simulink model "FirstOrder"  (R2020b)
settings: Solver=VariableStepAuto  StartTime=0.0  StopTime=100  RelTol=1e-3
settings Model: Creator=99003741  LastModifiedBy=99003741
settings SolverCC: AlgebraicLoopSolver=LineSearch

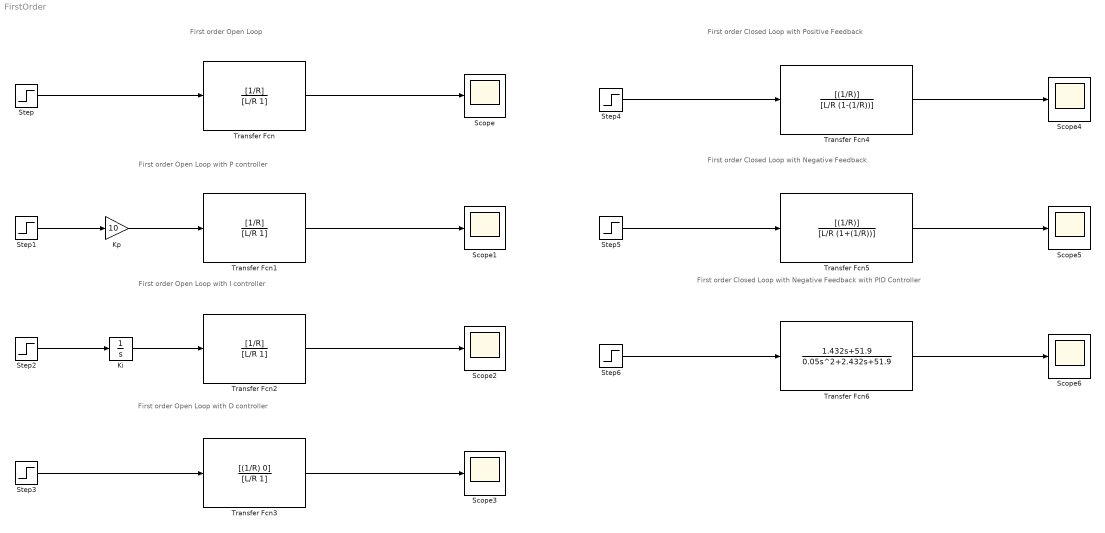
== system FirstOrder ==
  note: First order Open Loop
  note: First order Open Loop with P controller
  note: First order Open Loop with I controller
  note: First order Open Loop with D controller
  note: First order Closed Loop with Positive Feedback
  note: First order Closed Loop with Negative Feedback
  note: First order Closed Loop with Negative Feedback with PID Controller
  Ki : Integrator
  Kp : Gain  Gain=10
  Scope{,1..6} (7 alike) : Scope
  Step{,1..6} (7 alike) : Step  SampleTime=0
  Transfer Fcn : TransferFcn  Numerator=[1/R]  Denominator=[L/R 1]  mask{R=100, L=5}
  Transfer Fcn1 : TransferFcn  Numerator=[1/R]  Denominator=[L/R 1]  mask{R=100, L=5}
  Transfer Fcn2 : TransferFcn  Numerator=[1/R]  Denominator=[L/R 1]  mask{R=100, L=5}
  Transfer Fcn3 : TransferFcn  Numerator=[(1/R) 0]  Denominator=[L/R 1]  mask{R=100, L=5}
  Transfer Fcn4 : TransferFcn  Numerator=[(1/R)]  Denominator=[L/R (1-(1/R))]  mask{R=100, L=5}
  Transfer Fcn5 : TransferFcn  Numerator=[(1/R)]  Denominator=[L/R (1+(1/R))]  mask{R=100, L=5}
  Transfer Fcn6 : TransferFcn  Numerator=[1.432 51.9]  Denominator=[0.05 2.432 51.9]
  wires:
  Step/1 -> Transfer Fcn/1
  Transfer Fcn/1 -> Scope/1
  Transfer Fcn1/1 -> Scope1/1
  Step1/1 -> Kp/1
  Kp/1 -> Transfer Fcn1/1
  Transfer Fcn2/1 -> Scope2/1
  Step2/1 -> Ki/1
  Ki/1 -> Transfer Fcn2/1
  Transfer Fcn3/1 -> Scope3/1
  Step3/1 -> Transfer Fcn3/1
  Transfer Fcn4/1 -> Scope4/1
  Step4/1 -> Transfer Fcn4/1
  Step5/1 -> Transfer Fcn5/1
  Transfer Fcn5/1 -> Scope5/1
  Transfer Fcn6/1 -> Scope6/1
  Step6/1 -> Transfer Fcn6/1
